simulink model "quadcopter"  (R2021b)
settings: Solver=VariableStepAuto  StartTime=0.0  StopTime=10  RelTol=1e-3
values from neighbouring files (symbols this model uses):
  g = 9.806    [AccerationToEuler.m]
undefined symbols (not defined in the file or in its folder): arm_length, inertia_matrix, kf, mass, prop_breakpoints, prop_force, prop_moment
settings Model: Creator=hank2  LastModifiedBy=hank2

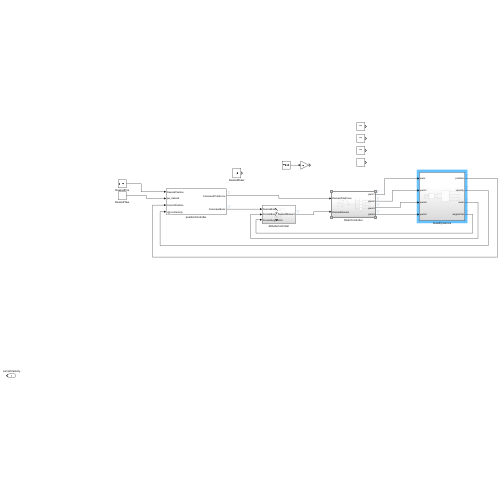
[thumbnail: Simulink's stored preview of the top-level diagram]
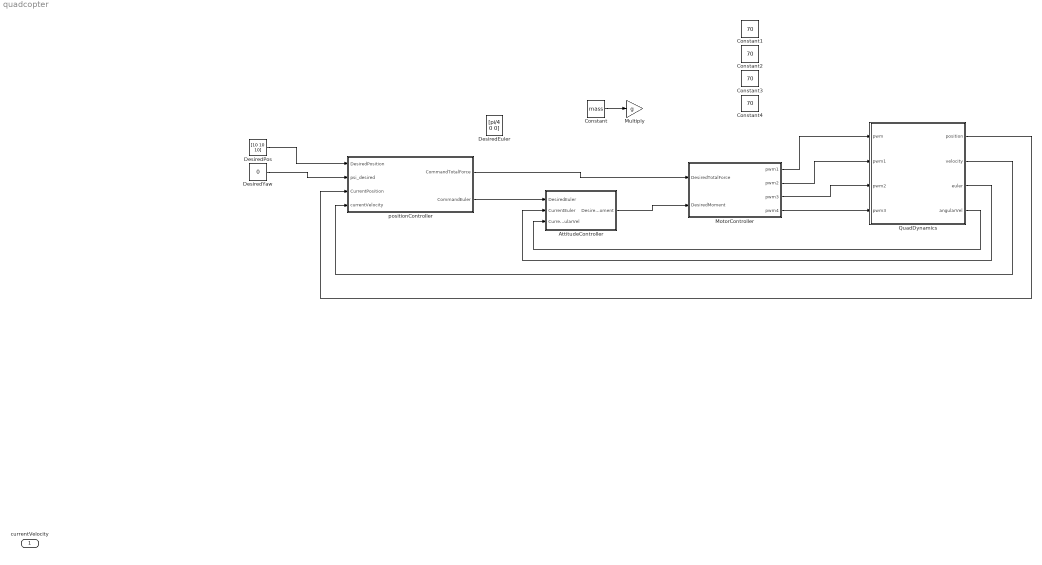
== system quadcopter ==
  currentVelocity : Inport
  AttitudeController : Subsystem
  Constant : Constant  Value=mass
  Constant{1..4} (4 alike) : Constant  Value=70
  DesiredEuler : Constant  Value=[pi/4 0 0]
  DesiredPos : Constant  Value=[10 10 10]
  DesiredYaw : Constant  Value=0
  MotorController : Subsystem
  Multiply : Gain  Gain=g
  QuadDynamics : Subsystem
  positionController : Subsystem  mask{mass=mass}
  wires:
  AttitudeController/1(DesiredMoment) -> MotorController/2(DesiredMoment)
  QuadDynamics/3(euler) -> AttitudeController/2(CurrentEuler)
  QuadDynamics/4(angularVel) -> AttitudeController/3(CurrentAngularVel)
  DesiredPos/1 -> positionController/1(DesiredPosition)
  DesiredYaw/1 -> positionController/2(psi_desired)
  Constant/1 -> Multiply/1
  MotorController/1(pwm1) -> QuadDynamics/1(pwm)
  MotorController/2(pwm2) -> QuadDynamics/2(pwm1)
  MotorController/3(pwm3) -> QuadDynamics/3(pwm2)
  MotorController/4(pwm4) -> QuadDynamics/4(pwm3)
  QuadDynamics/2(velocity) -> positionController/4(currentVelocity)
  QuadDynamics/1(position) -> positionController/3(CurrentPosition)
  positionController/1(CommandTotalForce) -> MotorController/1(DesiredTotalForce)
  positionController/2(CommandEuler) -> AttitudeController/1(DesiredEuler)

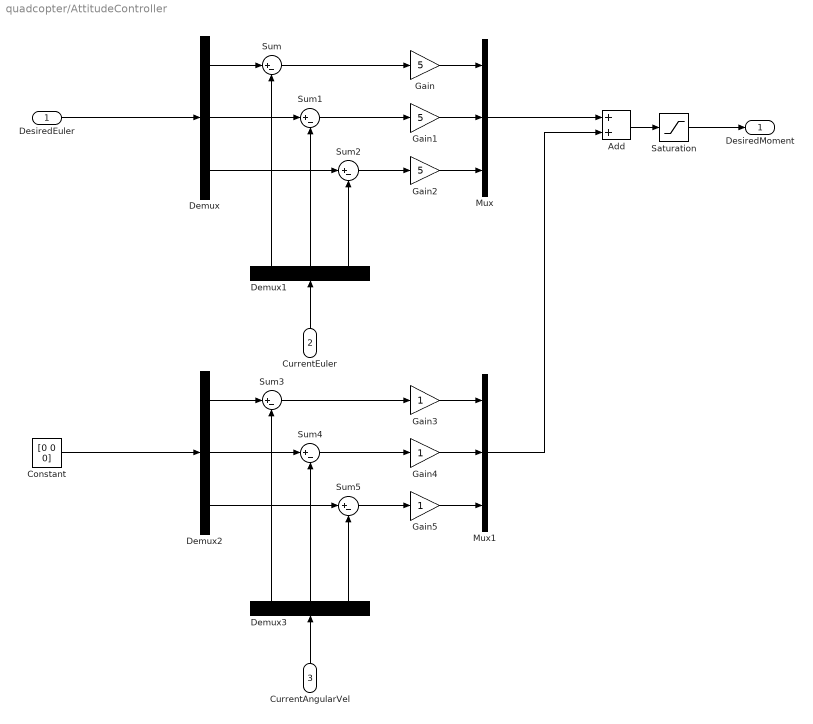
== system quadcopter/AttitudeController ==
  DesiredEuler : Inport  PortDimensions=3
  CurrentEuler : Inport  Port=2  PortDimensions=3
  CurrentAngularVel : Inport  Port=3  PortDimensions=3
  Add : Sum
  Constant : Constant  Value=[0 0 0]
  Demux{,1..3} (4 alike) : Demux  Outputs=3
  Gain : Gain  Gain=5
  Gain1 : Gain  Gain=5
  Gain2 : Gain  Gain=5
  Gain3 : Gain
  Gain4 : Gain
  Gain5 : Gain
  Mux : Mux  Inputs=3
  Mux1 : Mux  Inputs=3
  Saturation : Saturate  UpperLimit=4  LowerLimit=-4
  Sum{,1..5} (6 alike) : Sum  Inputs=|+-
  DesiredMoment : Outport  PortDimensions=3
  wires:
  Demux1/2 -> Sum1/2
  DesiredEuler/1 -> Demux/1
  CurrentEuler/1 -> Demux1/1
  Demux1/1 -> Sum/2
  Demux1/3 -> Sum2/2
  Demux/2 -> Sum1/1
  Demux/3 -> Sum2/1
  Demux/1 -> Sum/1
  Sum/1 -> Gain/1
  Gain/1 -> Mux/1
  Gain1/1 -> Mux/2
  Sum1/1 -> Gain1/1
  Gain2/1 -> Mux/3
  Sum2/1 -> Gain2/1
  Sum4/1 -> Gain4/1
  Gain4/1 -> Mux1/2
  CurrentAngularVel/1 -> Demux3/1
  Demux2/1 -> Sum3/1
  Demux2/3 -> Sum5/1
  Demux2/2 -> Sum4/1
  Demux3/2 -> Sum4/2
  Sum3/1 -> Gain3/1
  Sum5/1 -> Gain5/1
  Demux3/3 -> Sum5/2
  Gain3/1 -> Mux1/1
  Demux3/1 -> Sum3/2
  Gain5/1 -> Mux1/3
  Constant/1 -> Demux2/1
  Mux/1 -> Add/1
  Mux1/1 -> Add/2
  Add/1 -> Saturation/1
  Saturation/1 -> DesiredMoment/1

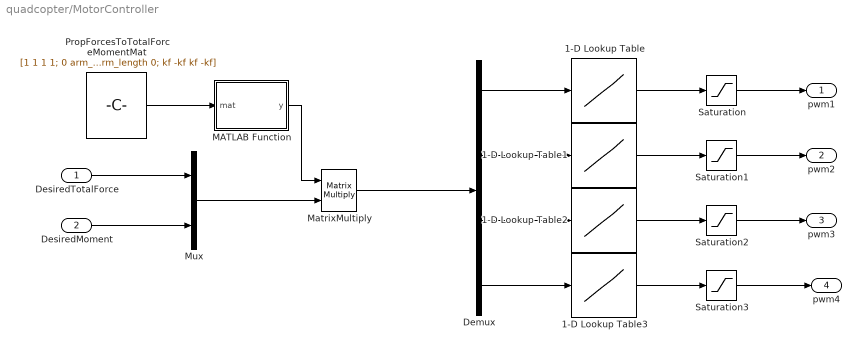
== system quadcopter/MotorController ==
  DesiredTotalForce : Inport
  DesiredMoment : Inport  Port=2
  1-D Lookup Table{,1..3} (4 alike) : Lookup_n-D  NumberOfTableDimensions=1  BreakpointsForDimension1=prop_force  Table=prop_breakpoints  InternalRulePriority=Speed  RndMeth=Simplest  InputSameDT=on
  Demux : Demux
  MATLAB Function : MATLAB Function  TreatAsAtomicUnit=on
  MatrixMultiply : Product  Multiplication=Matrix(*)
  Mux : Mux  Inputs=2
  PropForcesToTotalForceMomentMat : Constant  Value=[1 1 1 1; 0 arm_length 0 -arm_length; -arm_length 0 arm_length 0; kf -kf kf -kf]
  Saturation{,1..3} (4 alike) : Saturate  UpperLimit=100  LowerLimit=0
  pwm1 : Outport
  pwm2 : Outport  Port=2
  pwm3 : Outport  Port=3
  pwm4 : Outport  Port=4
  wires:
  Demux/4 -> 1-D Lookup Table3/1
  PropForcesToTotalForceMomentMat/1 -> MATLAB Function/1(mat)
  Demux/3 -> 1-D Lookup Table2/1
  MATLAB Function/1(y) -> MatrixMultiply/1
  Demux/1 -> 1-D Lookup Table/1
  Mux/1 -> MatrixMultiply/2
  Demux/2 -> 1-D Lookup Table1/1
  DesiredMoment/1 -> Mux/2
  DesiredTotalForce/1 -> Mux/1
  MatrixMultiply/1 -> Demux/1
  1-D Lookup Table/1 -> Saturation/1
  Saturation/1 -> pwm1/1
  1-D Lookup Table1/1 -> Saturation1/1
  1-D Lookup Table2/1 -> Saturation2/1
  Saturation2/1 -> pwm3/1
  1-D Lookup Table3/1 -> Saturation3/1
  Saturation3/1 -> pwm4/1
  Saturation1/1 -> pwm2/1

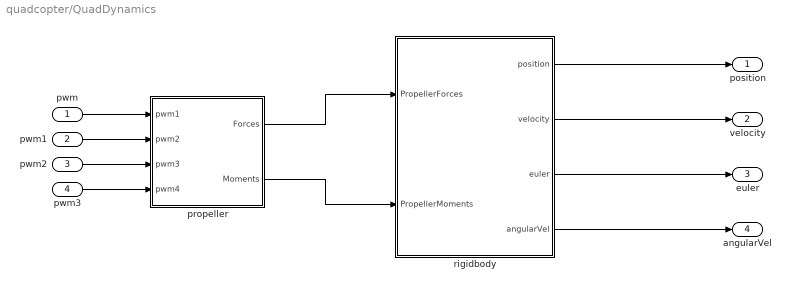
== system quadcopter/QuadDynamics ==
  pwm : Inport
  pwm1 : Inport  Port=2
  pwm2 : Inport  Port=3
  pwm3 : Inport  Port=4
  propeller : Subsystem
  rigidbody : Subsystem  mask{m=mass, L=arm_length, I=inertia_matrix, POS_INIT=[0 0 0], VEL_INIT=[0 0 0], EULER_INIT=[0 0 0], ANG_VEL_INIT=[0 0 0]}
      mask prompts: m "mass"; L "arm length"; I "Inertia Matrix"; POS_INIT "Initial Position (vector 3)"; VEL_INIT "Initial Velocity (vector 3)"; EULER_INIT "Initial Attitude (Roll Pitch Yaw)"; ANG_VEL_INIT "Initial Angular Velocity (vector 3)"
  position : Outport
  velocity : Outport  Port=2
  euler : Outport  Port=3
  angularVel : Outport  Port=4
  wires:
  rigidbody/3(euler) -> euler/1
  rigidbody/1(position) -> position/1
  rigidbody/4(angularVel) -> angularVel/1
  rigidbody/2(velocity) -> velocity/1
  pwm/1 -> propeller/1(pwm1)
  pwm1/1 -> propeller/2(pwm2)
  pwm2/1 -> propeller/3(pwm3)
  pwm3/1 -> propeller/4(pwm4)
  propeller/1(Forces) -> rigidbody/1(PropellerForces)
  propeller/2(Moments) -> rigidbody/2(PropellerMoments)

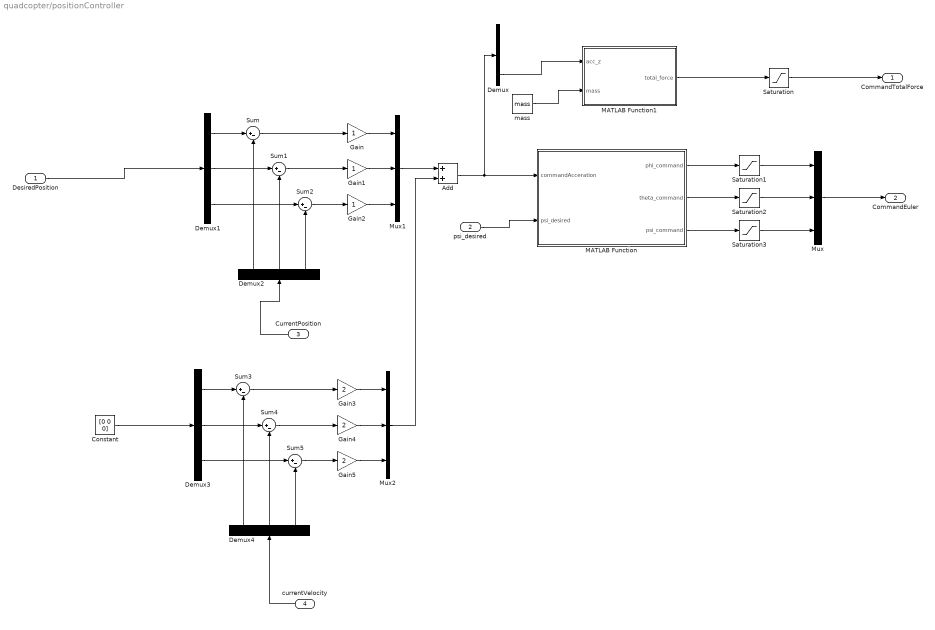
== system quadcopter/positionController ==
  DesiredPosition : Inport
  psi_desired : Inport  Port=2
  CurrentPosition : Inport  Port=3
  currentVelocity : Inport  Port=4
  Add : Sum
  Constant : Constant  Value=[0 0 0]
  Demux{,1..4} (5 alike) : Demux  Outputs=3
  Gain : Gain
  Gain1 : Gain
  Gain2 : Gain
  Gain3 : Gain  Gain=2
  Gain4 : Gain  Gain=2
  Gain5 : Gain  Gain=2
  MATLAB Function : MATLAB Function  TreatAsAtomicUnit=on
  MATLAB Function1 : MATLAB Function  TreatAsAtomicUnit=on
  Mux : Mux  Inputs=3
  Mux1 : Mux  Inputs=3
  Mux2 : Mux  Inputs=3
  Saturation : Saturate  UpperLimit=7  LowerLimit=0
  Saturation1 : Saturate  UpperLimit=pi/4  LowerLimit=-pi/4
  Saturation2 : Saturate  UpperLimit=pi/4  LowerLimit=-pi/4
  Saturation3 : Saturate  UpperLimit=pi/4  LowerLimit=-pi/4
  Sum{,1..5} (6 alike) : Sum  Inputs=|+-
  mass : Constant  Value=mass
  CommandTotalForce : Outport
  CommandEuler : Outport  Port=2
  wires:
  DesiredPosition/1 -> Demux1/1
  Sum3/1 -> Gain3/1
  Demux4/3 -> Sum5/2
  Demux2/2 -> Sum1/2
  CurrentPosition/1 -> Demux2/1
  Demux1/2 -> Sum1/1
  Constant/1 -> Demux3/1
  currentVelocity/1 -> Demux4/1
  Mux1/1 -> Add/1
  Demux3/1 -> Sum3/1
  Demux4/1 -> Sum3/2
  Mux2/1 -> Add/2
  Add/1 -> Demux/1, MATLAB Function/1(commandAcceration)
  Demux4/2 -> Sum4/2
  Sum4/1 -> Gain4/1
  Gain3/1 -> Mux2/1
  Demux2/1 -> Sum/2
  Demux1/1 -> Sum/1
  Gain5/1 -> Mux2/3
  Mux/1 -> CommandEuler/1
  Gain1/1 -> Mux1/2
  Sum5/1 -> Gain5/1
  psi_desired/1 -> MATLAB Function/2(psi_desired)
  Demux1/3 -> Sum2/1
  Demux/3 -> MATLAB Function1/1(acc_z)
  Demux3/3 -> Sum5/1
  Demux3/2 -> Sum4/1
  Gain4/1 -> Mux2/2
  Sum1/1 -> Gain1/1
  Sum2/1 -> Gain2/1
  Gain2/1 -> Mux1/3
  Demux2/3 -> Sum2/2
  Gain/1 -> Mux1/1
  Sum/1 -> Gain/1
  mass/1 -> MATLAB Function1/2(mass)
  Saturation/1 -> CommandTotalForce/1
  MATLAB Function1/1(total_force) -> Saturation/1
  Saturation1/1 -> Mux/1
  MATLAB Function/1(phi_command) -> Saturation1/1
  MATLAB Function/2(theta_command) -> Saturation2/1
  Saturation2/1 -> Mux/2
  MATLAB Function/3(psi_command) -> Saturation3/1
  Saturation3/1 -> Mux/3

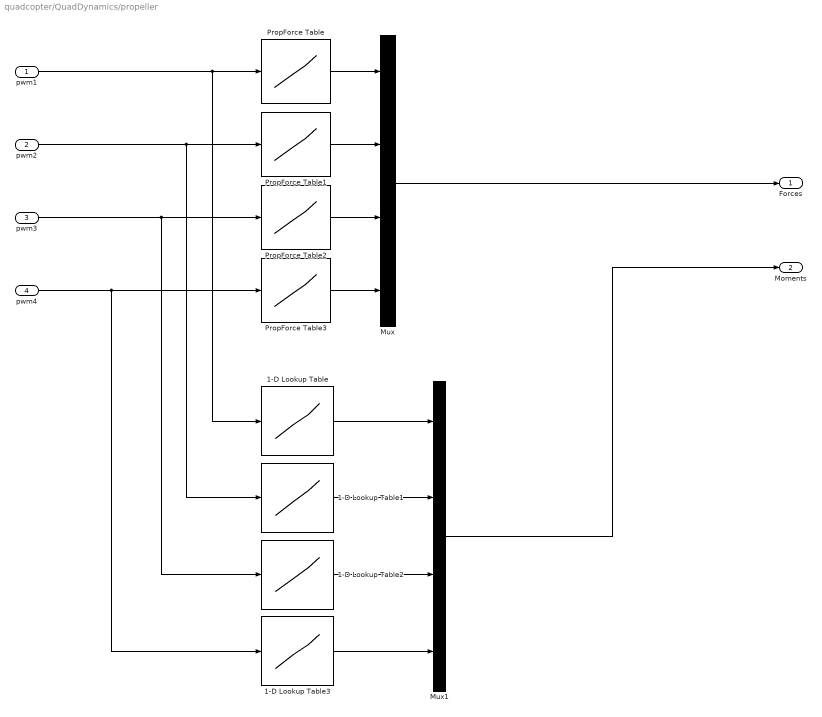
== system quadcopter/QuadDynamics/propeller ==
  pwm1 : Inport
  pwm2 : Inport  Port=2
  pwm3 : Inport  Port=3
  pwm4 : Inport  Port=4
  1-D Lookup Table{,1..3} (4 alike) : Lookup_n-D  NumberOfTableDimensions=1  BreakpointsForDimension1=prop_breakpoints  Table=prop_moment  InternalRulePriority=Speed  RndMeth=Simplest  InputSameDT=on
  Mux : Mux
  Mux1 : Mux
  PropForce Table{,1..3} (4 alike) : Lookup_n-D  NumberOfTableDimensions=1  BreakpointsForDimension1=prop_breakpoints  Table=prop_force  InternalRulePriority=Speed  RndMeth=Simplest  InputSameDT=on
  Forces : Outport
  Moments : Outport  Port=2
  wires:
  pwm2/1 -> 1-D Lookup Table1/1, PropForce Table1/1
  pwm1/1 -> 1-D Lookup Table/1, PropForce Table/1
  PropForce Table/1 -> Mux/1
  Mux/1 -> Forces/1
  1-D Lookup Table1/1 -> Mux1/2
  PropForce Table1/1 -> Mux/2
  pwm3/1 -> 1-D Lookup Table2/1, PropForce Table2/1
  1-D Lookup Table/1 -> Mux1/1
  1-D Lookup Table2/1 -> Mux1/3
  PropForce Table2/1 -> Mux/3
  pwm4/1 -> 1-D Lookup Table3/1, PropForce Table3/1
  1-D Lookup Table3/1 -> Mux1/4
  PropForce Table3/1 -> Mux/4
  Mux1/1 -> Moments/1

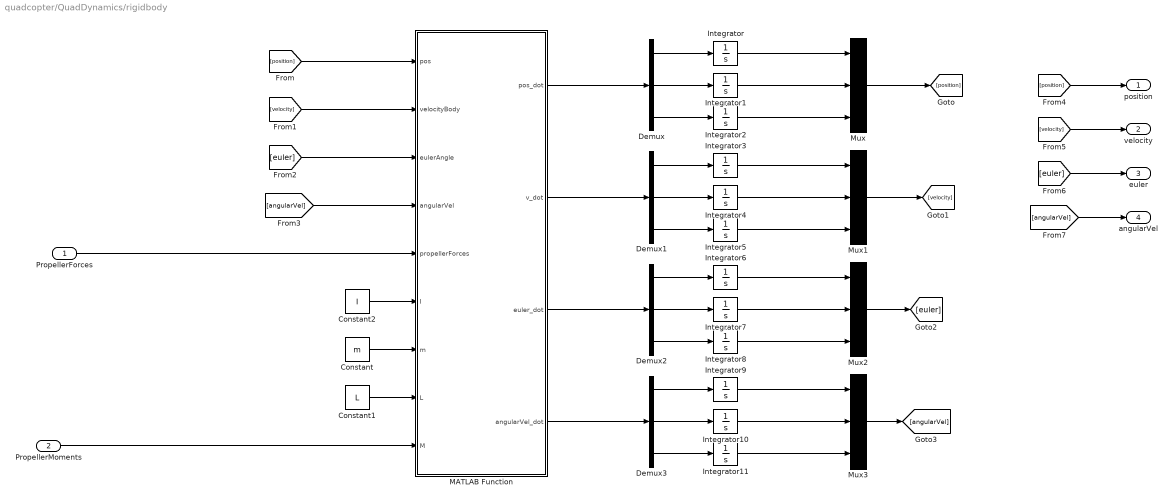
== system quadcopter/QuadDynamics/rigidbody ==
  PropellerForces : Inport  PortDimensions=4
  PropellerMoments : Inport  Port=2  PortDimensions=4
  Constant : Constant  Value=m
  Constant1 : Constant  Value=L
  Constant2 : Constant  Value=I
  Demux{,1..3} (4 alike) : Demux  Outputs=3
  Integrator : Integrator  InitialCondition=POS_INIT(1)
  Integrator1 : Integrator  InitialCondition=POS_INIT(2)
  Integrator10 : Integrator  InitialCondition=ANG_VEL_INIT(2)
  Integrator11 : Integrator  InitialCondition=ANG_VEL_INIT(3)
  Integrator2 : Integrator  InitialCondition=POS_INIT(3)
  Integrator3 : Integrator  InitialCondition=VEL_INIT(1)
  Integrator4 : Integrator  InitialCondition=VEL_INIT(2)
  Integrator5 : Integrator  InitialCondition=VEL_INIT(3)
  Integrator6 : Integrator  InitialCondition=EULER_INIT(1)
  Integrator7 : Integrator  InitialCondition=EULER_INIT(2)
  Integrator8 : Integrator  InitialCondition=EULER_INIT(3)
  Integrator9 : Integrator  InitialCondition=ANG_VEL_INIT(1)
  MATLAB Function : MATLAB Function  TreatAsAtomicUnit=on
  Mux{,1..3} (4 alike) : Mux  Inputs=3
  position : Outport
  velocity : Outport  Port=2
  euler : Outport  Port=3
  angularVel : Outport  Port=4
  wires:
  Mux2/1 -> [euler]
  Demux/1 -> Integrator/1
  Integrator6/1 -> Mux2/1
  Mux/1 -> [position]
  Integrator8/1 -> Mux2/3
  Mux3/1 -> [angularVel]
  PropellerForces/1 -> MATLAB Function/5(propellerForces)
  Integrator/1 -> Mux/1
  Constant1/1 -> MATLAB Function/8(L)
  [euler] -> euler/1
  Demux2/3 -> Integrator8/1
  Demux3/2 -> Integrator10/1
  Integrator5/1 -> Mux1/3
  Demux2/2 -> Integrator7/1
  Integrator7/1 -> Mux2/2
  Integrator1/1 -> Mux/2
  Integrator4/1 -> Mux1/2
  Integrator2/1 -> Mux/3
  [position] -> position/1
  Integrator11/1 -> Mux3/3
  Mux1/1 -> [velocity]
  Demux3/3 -> Integrator11/1
  Demux1/3 -> Integrator5/1
  Demux/2 -> Integrator1/1
  Demux3/1 -> Integrator9/1
  Integrator3/1 -> Mux1/1
  Integrator9/1 -> Mux3/1
  Demux2/1 -> Integrator6/1
  Demux1/2 -> Integrator4/1
  Demux/3 -> Integrator2/1
  Demux1/1 -> Integrator3/1
  PropellerMoments/1 -> MATLAB Function/9(M)
  Integrator10/1 -> Mux3/2
  [angularVel] -> angularVel/1
  [velocity] -> velocity/1
  Constant/1 -> MATLAB Function/7(m)
  Constant2/1 -> MATLAB Function/6(I)
  [angularVel] -> MATLAB Function/4(angularVel)
  [velocity] -> MATLAB Function/2(velocityBody)
  [euler] -> MATLAB Function/3(eulerAngle)
  [position] -> MATLAB Function/1(pos)
  MATLAB Function/1(pos_dot) -> Demux/1
  MATLAB Function/2(v_dot) -> Demux1/1
  MATLAB Function/4(angularVel_dot) -> Demux3/1
  MATLAB Function/3(euler_dot) -> Demux2/1

== matlab function quadcopter/MotorController/MATLAB Function ==
  data: mat input; y output
function y = inverse(mat)
    y = inv(mat);
end

== matlab function quadcopter/QuadDynamics/rigidbody/MATLAB Function ==
  data: pos input; velocityBody input; eulerAngle input; angularVel input; pos_dot output; propellerForces input; I input; m input; L input; M input; v_dot output; euler_dot output; angularVel_dot output
% x = x y z u v w phi theta psi p q r
% input = F1 F2 F3 F4
% I inertia matrix
% m mass
% L quad arm length
% M moments of each propeller
function [pos_dot, v_dot, euler_dot, angularVel_dot] = quadDyanmics(pos, velocityBody, eulerAngle, angularVel, propellerForces, I, m, L, M)
%   specify output size
    pos_dot = zeros(3,1);
    v_dot = zeros(3,1);
    euler_dot = zeros(3,1);
    angularVel_dot = zeros(3,1);
    
    g = 9.806;
    F1 = propellerForces(1);
    F2 = propellerForces(2);
    F3 = propellerForces(3);
    F4 = propellerForces(4);
    phi = eulerAngle(1);
    theta = eulerAngle(2);
    psi = eulerAngle(3);
    Rz = [cos(psi) -sin(psi) 0;
          sin(psi) cos(psi)  0;
          0        0         1];
    Ry = [cos(theta)  0 sin(theta);
          0           1          0;
          -sin(theta) 0 cos(theta)];
    Rx = [1 0                0;
          0 cos(phi) -sin(phi);
          0 sin(phi)  cos(phi)];
    R = Rz*Ry*Rx;
%     differential equation
    pos_dot = R*velocityBody;
    v_dot = R'*[0 0 -g]' + [0 0 (F1 + F2 + F3 + F4)/m]';
    euler_dot = [1 sin(phi)*tan(theta) cos(phi)*tan(theta);
                 0 cos(phi)            -sin(phi);
                 0 sin(phi)*sec(theta) cos(phi)*sec(theta)]*angularVel;
    angularVel_dot = inv(I)*([L*(F2-F4); ...
                              L*(F3-F1); ...
                              M(1)-M(2)+M(3)-M(4)] ...
                              - cross(angularVel,I*angularVel));
    
end

== matlab function quadcopter/positionController/MATLAB Function ==
  data: commandAcceration input; phi_command output; psi_desired input; theta_command output; psi_command output
function [phi_command, theta_command, psi_command] = AcceerationToEuler(commandAcceration, psi_desired)
    g = 9.806;
    accx_desire = commandAcceration(1); 
    accy_desire = commandAcceration(2); 
    accz_desire = commandAcceration(3);
    eulerToAccMat = g*[sin(psi_desired) cos(psi_desired);...
                       -cos(psi_desired) sin(psi_desired)];
    command_phi_theta = inv(eulerToAccMat)*[accx_desire;accy_desire];
    phi_command = command_phi_theta(1);
    theta_command = command_phi_theta(2);
    psi_command = psi_desired;
end

== matlab function quadcopter/positionController/MATLAB Function1 ==
  data: acc_z input; total_force output; mass input
function total_force = calculateTotalForce(acc_z, mass)
    g = 9.806;
    total_force = mass*(g + acc_z);
end
